simulink model "starterProject03"  (R2020b)
settings: Solver=ode1  StartTime=0.0  StopTime=inf  FixedStep=0.001  RelTol=1e-3  EnableMultiTasking=on
libraries: arduinolib x2
settings Model: SimulationMode=external  SILPILModeSetting=veronly  ExtModeTrigDuration=2  Creator=kitaw  LastModifiedBy=kitaw
settings DataIOCC: ReturnWorkspaceOutputs=off
settings OptimizationCC: MaxStackSize=64
settings DebuggingCC: ParameterTunabilityLossMsg=error  ArithmeticOperatorsInVariantConditions=warning
settings HardwareCC: ProdBitPerInt=16  ProdBitPerPointer=16  ProdBitPerSizeT=16  ProdBitPerPtrDiffT=16  ProdLargestAtomicFloat=None  ProdWordSize=8  ProdHWDeviceType=Atmel->AVR  UseEmbeddedCoderFeatures=off  UseSimulinkCoderFeatures=off
settings SFSimCC: SimUseLocalCustomCode=off  CustomCodeUndefinedFunction=UseInterfaceOnly
settings RTWCC: Description=Embedded Coder  SystemTargetFile=ert.tlc  HardwareBoard=Arduino Uno  TemplateMakefile=ert_default_tmf  GenerateReport=on  RTWUseLocalCustomCode=off  Toolchain=Arduino AVR  BuildConfiguration=Faster Runs  LaunchReport=on
settings CodeAppCC: ForceParamTrailComments=on  OperatorAnnotations=on  StateflowObjectComments=on  MATLABSourceComments=on
settings ERTTargetCC: ERTCustomFileBanners=off  SupportContinuousTime=on  SupportNonInlinedSFcns=on  RemoveResetFunc=off  SupportVariableSizeSignals=on  ModelStepFunctionPrototypeControlCompliant=off  ExtModeStaticAllocSize=250

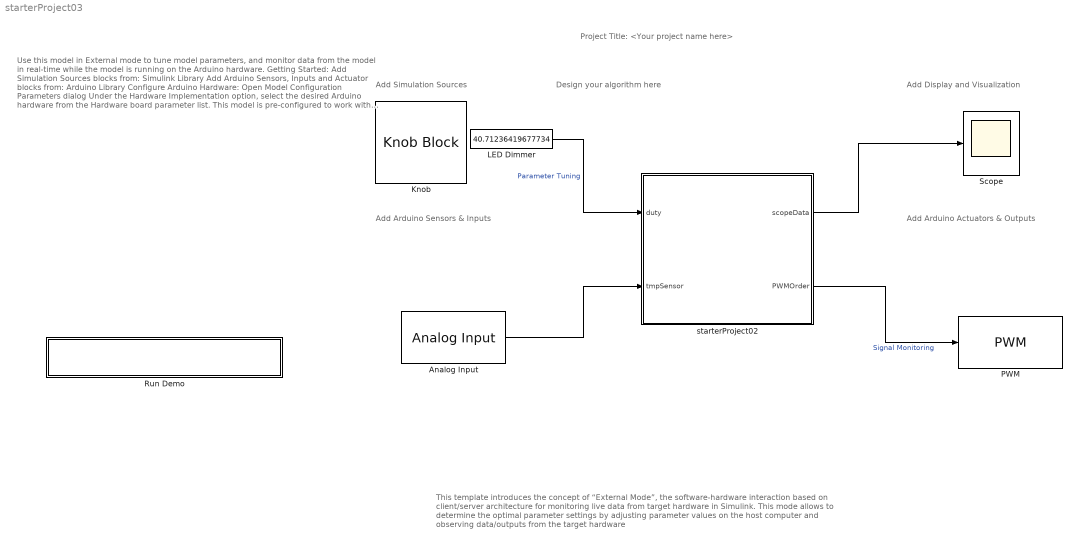
== system starterProject03 ==
  note: Project Title: <Your project name here>
  note: Use this model in External mode to tune model parameters, and monitor data from the model in real-time while the model is running on the Arduino hardware.
      |
      | Getting Started:
      |
      | Add Simulation Sources blocks from:
      | Simulink Library
      | Add Arduino Sensors, Inputs and Actuator blocks from:
      | Arduino Library
      |
      | Configure Arduino Hardware:
      |
      | Open Model Configuration Parameters dialog
      | Under the Hardware Implementation option, select the desired Arduino hardware from the Hardware board parameter list.
      |
      | This model is pre-configured to work with Arduino Mega 2560.
      |
      | Run the Model on Arduino Hardware (External Mode)
      |
      | On the Simulink Editor toolbar, set simulation mode to External
      |
      | External mode will stop when the number of seconds specified in the Simulation stop time parameter elapses.
      |
      | Learn More:
      |
      | Tune and Monitor Model Running on Arduino Mega 2560 Hardware
  note: Add Display and Visualization
  note: Add Arduino Sensors & Inputs
  note: Design your algorithm here
  note: Add Simulation Sources
  note: Add Arduino Actuators & Outputs
  note: This template introduces the concept of “External Mode”, the software-hardware interaction based on client/server architecture for monitoring live data from target hardware in Simulink. This mode allows to determine the optimal parameter settings by adjusting parameter values on the host computer and observing data/outputs from the target hardware
  Analog Input : arduinolib/Analog Input  pinNumber=0  ReadResultsOnly=off  ConversionTriggerSource=Software  ExternalTriggerType=uint32(0)  OutputDataType=uint16  EnableConversionCompleteNotify=off  EnableOuputStatus=off  SampleTime=-1  blockPlatform=arduino
  Knob : KnobBlock  TickInterval=10
  LED Dimmer : Constant  Value=40.71236419677734  OutDataTypeStr=uint8  SampleTime=0.1
  PWM : arduinolib/PWM  pinNumber=3  frequencyType=Default  desiredFrequency=490.2  achievableFrequency=490.2
  Run Demo : Subsystem  Description=Controls host-side RTDX processing.
      mask Display: pic=imread('arduinoExternalMode.png');image(pic);
  Scope : Scope
  starterProject02 : Subsystem
  wires:
  LED Dimmer/1 -> starterProject02/1(duty)  "Parameter Tuning"
  Analog Input/1 -> starterProject02/2(tmpSensor)
  starterProject02/1(scopeData) -> Scope/1
  starterProject02/2(PWMOrder) -> PWM/1  "Signal Monitoring"

== system starterProject03/Run Demo ==

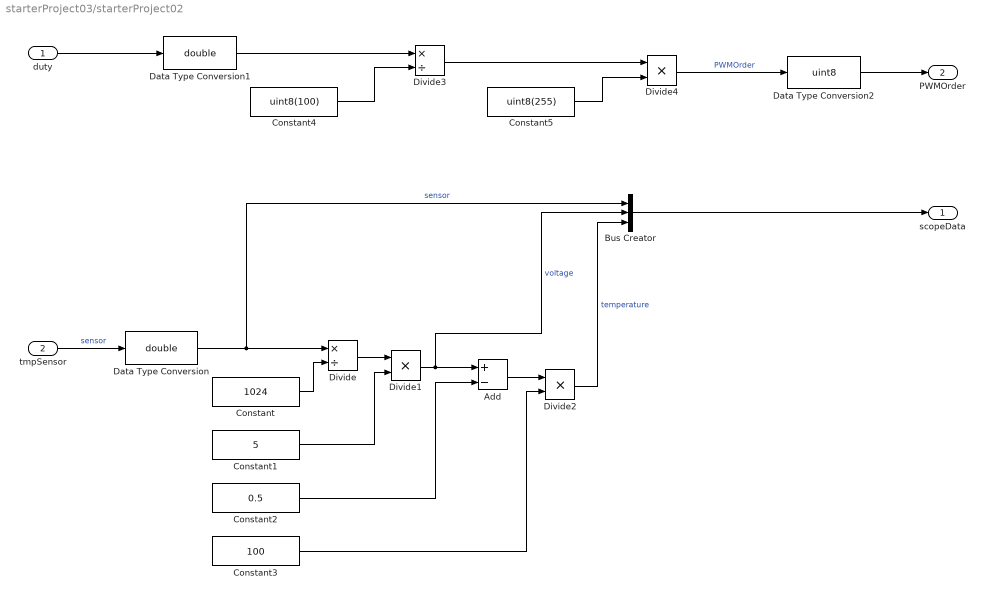
== system starterProject03/starterProject02 ==
  duty : Inport
  tmpSensor : Inport  Port=2
  Add : Sum  Inputs=+-
  Bus Creator : BusCreator  Inputs=3
  Constant : Constant  Value=1024
  Constant1 : Constant  Value=5
  Constant2 : Constant  Value=0.5
  Constant3 : Constant  Value=100
  Constant4 : Constant  Value=uint8(100)
  Constant5 : Constant  Value=uint8(255)
  Data Type Conversion : DataTypeConversion  OutDataTypeStr=double
  Data Type Conversion1 : DataTypeConversion  OutDataTypeStr=double
  Data Type Conversion2 : DataTypeConversion  OutDataTypeStr=uint8
  Divide : Product  Inputs=*/
  Divide1 : Product  Inputs=**
  Divide2 : Product  Inputs=**
  Divide3 : Product  Inputs=*/
  Divide4 : Product  Inputs=**
  scopeData : Outport  VectorParamsAs1DForOutWhenUnconnected=off
  PWMOrder : Outport  Port=2  VectorParamsAs1DForOutWhenUnconnected=off
  wires:
  Bus Creator/1 -> scopeData/1
  tmpSensor/1 -> Data Type Conversion/1  "sensor"
  Constant/1 -> Divide/2
  Divide/1 -> Divide1/1
  Constant1/1 -> Divide1/2
  Divide1/1 -> Add/1, Bus Creator/2  "voltage"
  Constant2/1 -> Add/2
  Add/1 -> Divide2/1
  Constant3/1 -> Divide2/2
  Divide2/1 -> Bus Creator/3  "temperature"
  Constant4/1 -> Divide3/2
  duty/1 -> Data Type Conversion1/1
  Divide3/1 -> Divide4/1
  Constant5/1 -> Divide4/2
  Divide4/1 -> Data Type Conversion2/1  "PWMOrder"
  Data Type Conversion/1 -> Bus Creator/1, Divide/1  "sensor"
  Data Type Conversion1/1 -> Divide3/1
  Data Type Conversion2/1 -> PWMOrder/1
